simulink model "DifferenceEquation"  (R2020b)
settings: Solver=VariableStepAuto  StartTime=0.0  StopTime=0.1  RelTol=1e-3
settings Model: Creator=Training  LastModifiedBy=Training

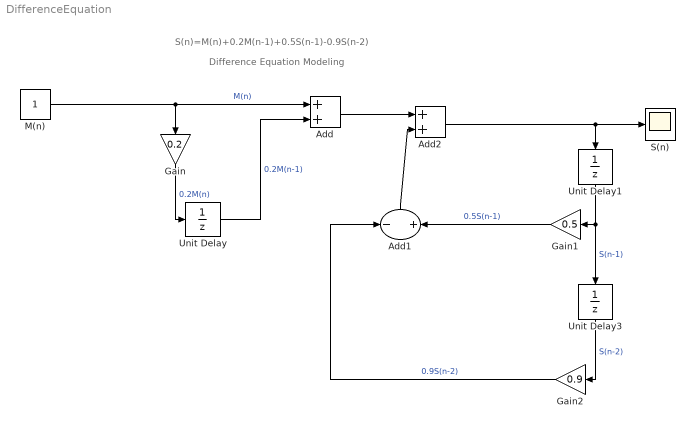
== system DifferenceEquation ==
  note: Difference Equation Modeling
  note: S(n)=M(n)+0.2M(n-1)+0.5S(n-1)-0.9S(n-2)
  Add : Sum
  Add1 : Sum  Inputs=-+
  Add2 : Sum
  Gain : Gain  Gain=0.2
  Gain1 : Gain  Gain=0.5
  Gain2 : Gain  Gain=0.9
  M(n) : Constant
  S(n) : Scope
  Unit Delay : UnitDelay  SampleTime=-1  HasFrameUpgradeWarning=on
  Unit Delay1 : UnitDelay  SampleTime=-1  HasFrameUpgradeWarning=on
  Unit Delay3 : UnitDelay  SampleTime=-1  HasFrameUpgradeWarning=on
  wires:
  M(n)/1 -> Add/1, Gain/1  "M(n)"
  Gain/1 -> Unit Delay/1  "0.2M(n)"
  Unit Delay/1 -> Add/2  "0.2M(n-1)"
  Unit Delay1/1 -> Unit Delay3/1, Gain1/1  "S(n-1)"
  Unit Delay3/1 -> Gain2/1  "S(n-2)"
  Add/1 -> Add2/1
  Add2/1 -> Unit Delay1/1, S(n)/1
  Add1/1 -> Add2/2
  Gain1/1 -> Add1/2  "0.5S(n-1)"
  Gain2/1 -> Add1/1  "0.9S(n-2)"
